simulink model "Problem_3"  (R2020b)
settings: Solver=VariableStepAuto  StartTime=0.0  StopTime=180  RelTol=1e-3
values from neighbouring files (symbols this model uses):
  b = 50    [parameters.m]
  Ki = 40    [parameters.m]
  Kp = 800    [parameters.m]
  m = 1000    [parameters.m]
settings Model: Creator=adity  LastModifiedBy=adity

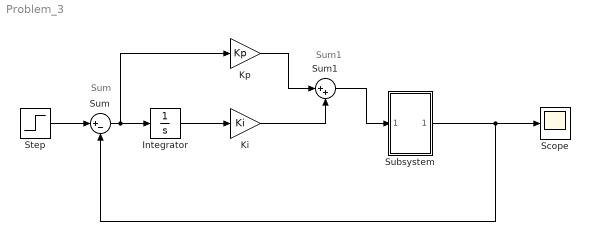
== system Problem_3 ==
  note: Sum1
  note: Sum
  Integrator : Integrator
  Ki : Gain  Gain=Ki
  Kp : Gain  Gain=Kp
  Scope : Scope
  Step : Step  Time=0  After=u  SampleTime=0
  Subsystem : Subsystem
  Sum : Sum  Inputs=|+-
  Sum1 : Sum  Inputs=|++
  wires:
  Subsystem/1(Out1) -> Scope/1, Sum/2
  Integrator/1 -> Ki/1
  Step/1 -> Sum/1
  Ki/1 -> Sum1/2
  Sum/1 -> Kp/1, Integrator/1
  Kp/1 -> Sum1/1
  Sum1/1 -> Subsystem/1(In1)

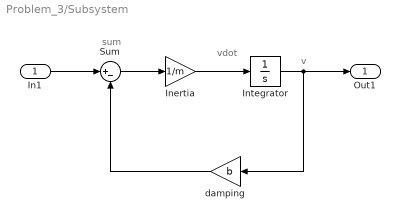
== system Problem_3/Subsystem ==
  note: sum
  note: vdot
  note: v
  In1 : Inport
  Inertia : Gain  Gain=1/m
  Integrator : Integrator
  Sum : Sum  Inputs=|+-
  damping : Gain  Gain=b
  Out1 : Outport
  wires:
  In1/1 -> Sum/1
  Sum/1 -> Inertia/1
  Inertia/1 -> Integrator/1
  damping/1 -> Sum/2
  Integrator/1 -> Out1/1, damping/1
